simulink model "3D Inverted x-y Pendulum Modeling"  (R2023b)
settings: Solver=VariableStepAuto  StartTime=0.0  StopTime=15  RelTol=1e-3
libraries: simulink x4
settings Model: Creator=Hamid Reza  LastModifiedBy=Hamid Reza

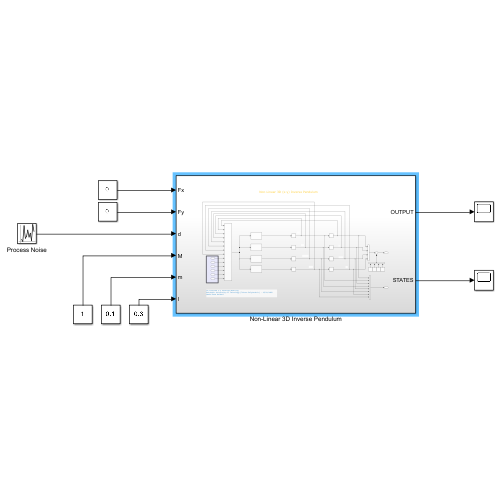
[thumbnail: Simulink's stored preview of the top-level diagram]
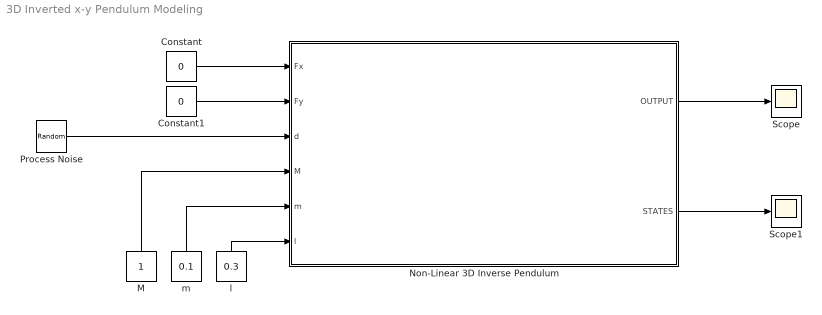
== system 3D Inverted x-y Pendulum Modeling ==
  Constant : Constant  Value=0
  Constant1 : Constant  Value=0
  M : Constant
  Non-Linear 3D Inverse Pendulum : Subsystem
  Process Noise : UniformRandomNumber  Minimum=-5  Maximum=5  Seed=1  SampleTime=0.1
  Scope : Scope
  Scope1 : Scope
  l : Constant  Value=0.3
  m : Constant  Value=0.1
  wires:
  l/1 -> Non-Linear 3D Inverse Pendulum/6(l)
  m/1 -> Non-Linear 3D Inverse Pendulum/5(m)
  M/1 -> Non-Linear 3D Inverse Pendulum/4(M)
  Constant1/1 -> Non-Linear 3D Inverse Pendulum/2(Fy)
  Constant/1 -> Non-Linear 3D Inverse Pendulum/1(Fx)
  Process Noise/1 -> Non-Linear 3D Inverse Pendulum/3(d)
  Non-Linear 3D Inverse Pendulum/1(OUTPUT) -> Scope/1
  Non-Linear 3D Inverse Pendulum/2(STATES) -> Scope1/1

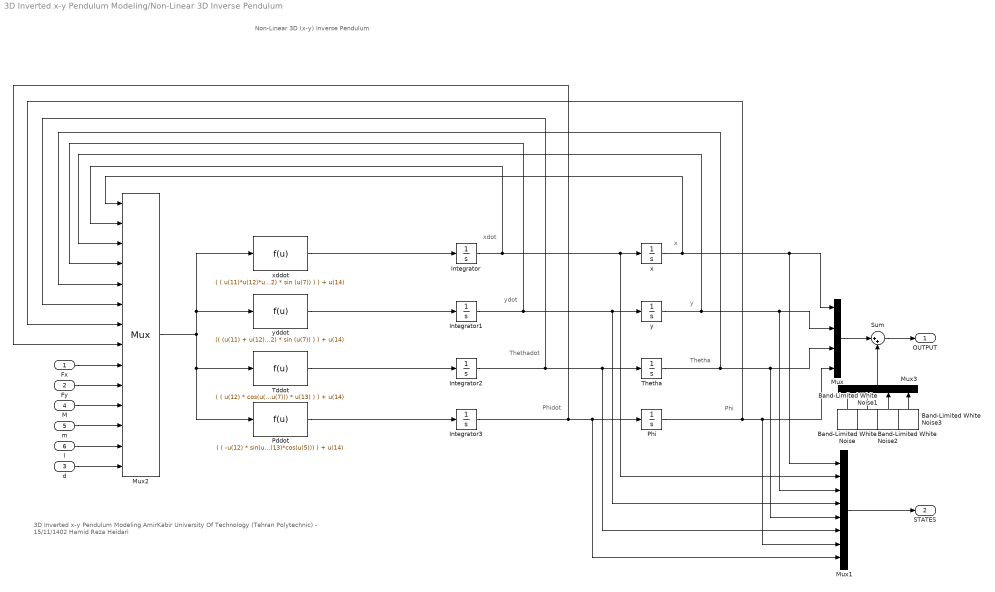
== system 3D Inverted x-y Pendulum Modeling/Non-Linear 3D Inverse Pendulum ==
  note: Non-Linear 3D (x-y) Inverse Pendulum
  note: 3D Inverted x-y Pendulum Modeling
      | AmirKabir University Of Technology (Tehran Polytechnic) - 15/11/1402
      | Hamid Reza Heidari
  note: xdot
  note: ydot
  note: Thethadot
  note: Phidot
  note: x
  note: y
  note: Thetha
  note: Phi
  Fx : Inport
  Fy : Inport  Port=2
  d : Inport  Port=3
  M : Inport  Port=4
  m : Inport  Port=5
  l : Inport  Port=6
  Band-Limited White Noise : simulink/Sources/Band-Limited White Noise  Cov=[0.1]  Ts=0.1  seed=[23341]
  Band-Limited White Noise1 : simulink/Sources/Band-Limited White Noise  Cov=[0.1]  Ts=0.1  seed=[23340]
  Band-Limited White Noise2 : simulink/Sources/Band-Limited White Noise  Cov=[0.1]  Ts=0.1  seed=[23339]
  Band-Limited White Noise3 : simulink/Sources/Band-Limited White Noise  Cov=[0.1]  Ts=0.1  seed=[23338]
  Integrator{,1..3} (4 alike) : Integrator
  Mux : Mux
  Mux1 : Mux  Inputs=8
  Mux2 : Mux  Inputs=14
  Mux3 : Mux
  Pddot : Fcn  Expr=|
      | ( ( -u(12) * sin(u(5))^2 * cos(u(7)) * u(10) - u(11) * cos(u(7)) * u(10) + u(12) * sin(u(5)) * cos(u(5)) * sin(u(7)) * cos(u(7)) * u(9) + 2*u(11)*u(12)*u(13) * sin(u(5)*u(6)*u(8)) + u(11)*(u(12) + u(11))*9.81 * sin (u(7)) + 2*(u(11)^2)*u(13) * sin (u(5)*u(6)*u(8))
      | - 2 * u(11)*u(12)*u(13) * sin(u(5)) * cos(u(5))^2 * cos(u(7)*u(6)*u(8))^2 - u(11)*u(12)*u(13) * cos(u(5))^3 * sin (u(7)) * cos (u(7)*(u(8)^2)) - u(11)*u(12)*u(13) * cos(u(5)) * sin(u(7)) * cos(u(7)*(u(6)^2)) ) / ( (u(11)^2+u(11)*u(12) * sin(u(5))^2 * cos(u(7))^2 +u(11)*u(12) * sin (u(7)))*u(13)*cos(u(5))) ) + u(14)
  Phi : Integrator
  Sum : Sum  Inputs=|++
  Tddot : Fcn  Expr=|
      | ( ( u(12) * cos(u(5)) * cos(u(7))^2 * u(9) - (u(11) + u(12)) * cos(u(5)) * u(9) + (u(11) + u(12)) * sin(u(5)) * sin(u(7)) * u(10) + u(11)*(u(12) + u(11))*9.81 * sin(u(5)) * cos(u(7))
      | - u(11)*u(12)*u(13) * sin(u(5)) * cos (u(5)) * cos (u(7)*(u(6)^2))^2 - u(11)*(u(12) + u(11))*u(13) * cos(u(5)) * sin(u(7)*(u(8)^2))  ) / ( (u(11)^2+u(11)*u(12) * sin(u(5))^2 * cos(u(7))^2 +u(11)*u(12) * sin (u(7))) * u(13) ) ) + u(14)
  Thetha : Integrator
  x : Integrator
  xddot : Fcn  Expr=|
      | ( ( u(11)*u(12)*u(13)* (sin(u(5)*(u(6)^2))) + u(11)*u(12)*u(13) * (cos(u(5)))^2 * (sin(u(5)*(u(8)^2))) - u(11)*u(12)*9.81 * (cos(u(5)))^2 * sin(u(5)) * cos(u(7))^2
      | + u(12) * cos(u(5))^2 * sin(u(7))^2 * u(9) + u(11) * u(9) - u(12) * cos(u(5))^2 * sin (u(5)) * sin (u(7)) * u(10) ) / ( u(11)^2+u(11)*u(12) * sin(u(5))^2 * cos(u(7))^2 +u(11)*u(12) * sin (u(7)) ) ) + u(14)
  y : Integrator
  yddot : Fcn  Expr=|
      | (( (u(11) + u(12)) * u(10) - u(12) * cos (u(5))^2 * u(10) + u(12) * sin (u(5)) * cos(u(5)) * sin (u(7)) * u(9) - u(11)*u(12)*9.81 * cos(u(5))^2 * sin (u(7)) * cos (u(7)) + u(11)*u(12)*u(13) * cos(u(5))^3 * sin (u(7)*(u(8)^2)) - u(11)*u(12)*u(13) * cos (u(5)) * sin (u(7)*(u(6)^2)) ) / ( u(11)^2+u(11)*u(12) * sin(u(5))^2 * cos(u(7))^2 +u(11)*u(12) * sin (u(7)) )
      | ) + u(14)
  OUTPUT : Outport
  STATES : Outport  Port=2
  wires:
  Mux2/1 -> Tddot/1, Pddot/1, xddot/1, yddot/1
  Integrator/1 -> Mux1/2, x/1, Mux2/2
  Integrator1/1 -> Mux2/4, Mux1/4, y/1
  Integrator2/1 -> Mux2/6, Mux1/6, Thetha/1
  Integrator3/1 -> Mux2/8, Mux1/8, Phi/1
  xddot/1 -> Integrator/1
  yddot/1 -> Integrator1/1
  Tddot/1 -> Integrator2/1
  Pddot/1 -> Integrator3/1
  Fx/1 -> Mux2/9
  Fy/1 -> Mux2/10
  M/1 -> Mux2/11
  m/1 -> Mux2/12
  l/1 -> Mux2/13
  d/1 -> Mux2/14
  x/1 -> Mux1/1, Mux/1, Mux2/1
  y/1 -> Mux1/3, Mux/2, Mux2/3
  Thetha/1 -> Mux2/5, Mux1/5, Mux/3
  Phi/1 -> Mux1/7, Mux/4, Mux2/7
  Mux1/1 -> STATES/1
  Sum/1 -> OUTPUT/1
  Mux/1 -> Sum/1
  Mux3/1 -> Sum/2
  Band-Limited White Noise/1 -> Mux3/1
  Band-Limited White Noise3/1 -> Mux3/4
  Band-Limited White Noise1/1 -> Mux3/2
  Band-Limited White Noise2/1 -> Mux3/3
